simulink library "Brown_Sensors_lib"  (R2025b)
settings: Solver=VariableStepAuto  StartTime=0.0  StopTime=10.0  RelTol=1e-3
undefined symbols (not defined in the file or in its folder): default_sensor_gps_cfg, default_sensor_scalar_cfg, default_sensor_vec3_cfg, sensor_scalar_block_step, sensor_vector3_block_step
settings Model: Creator=zbrown  LastModifiedBy=zbrown

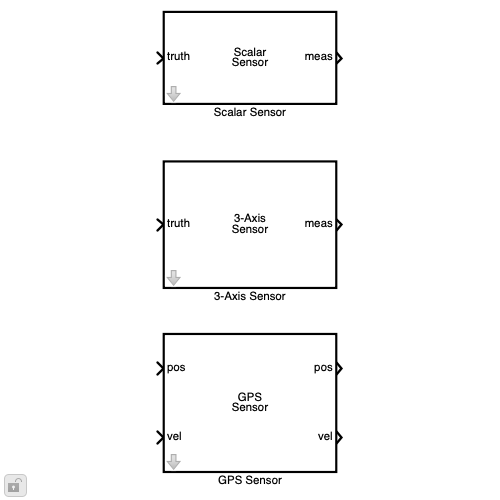
[thumbnail: Simulink's stored preview of the top-level diagram]
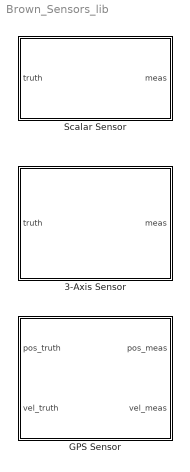
== system Brown_Sensors_lib ==
  3-Axis Sensor : Subsystem  TreatAsAtomicUnit=on  mask{cfg=default_sensor_vec3_cfg()}
      mask help: Simple reusable sensor model block.
      mask Display:
      | color('black');
      | disp('3-Axis\nSensor');
      | port_label('input',1,'truth');
      | port_label('output',1,'meas');
  GPS Sensor : Subsystem  TreatAsAtomicUnit=on  mask{cfg=default_sensor_gps_cfg()}
      mask help: Simple reusable sensor model block.
      mask Display:
      | color('black');
      | disp('GPS\nSensor');
      | port_label('input',1,'pos');
      | port_label('input',2,'vel');
      | port_label('output',1,'pos');
      | port_label('output',2,'vel');
  Scalar Sensor : Subsystem  TreatAsAtomicUnit=on  mask{cfg=default_sensor_scalar_cfg()}
      mask help: Simple reusable sensor model block.
      mask Display:
      | color('black');
      | disp('Scalar\nSensor');
      | port_label('input',1,'truth');
      | port_label('output',1,'meas');

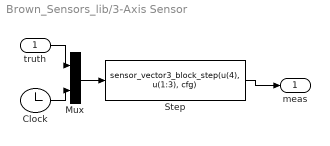
== system Brown_Sensors_lib/3-Axis Sensor ==
  truth : Inport  PortDimensions=3
  Clock : Clock
  Mux : Mux  Inputs=2
  Step : MATLABFcn  MATLABFcn=sensor_vector3_block_step(u(4), u(1:3), cfg)
  meas : Outport  PortDimensions=3
  wires:
  truth/1 -> Mux/1
  Clock/1 -> Mux/2
  Mux/1 -> Step/1
  Step/1 -> meas/1

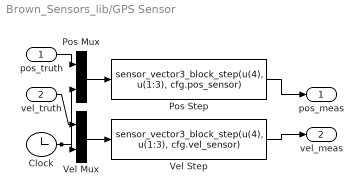
== system Brown_Sensors_lib/GPS Sensor ==
  pos_truth : Inport  PortDimensions=3
  vel_truth : Inport  Port=2  PortDimensions=3
  Clock : Clock
  Pos Mux : Mux  Inputs=2
  Pos Step : MATLABFcn  MATLABFcn=sensor_vector3_block_step(u(4), u(1:3), cfg.pos_sensor)
  Vel Mux : Mux  Inputs=2
  Vel Step : MATLABFcn  MATLABFcn=sensor_vector3_block_step(u(4), u(1:3), cfg.vel_sensor)
  pos_meas : Outport  PortDimensions=3
  vel_meas : Outport  Port=2  PortDimensions=3
  wires:
  pos_truth/1 -> Pos Mux/1
  Clock/1 -> Pos Mux/2, Vel Mux/2
  Pos Mux/1 -> Pos Step/1
  vel_truth/1 -> Vel Mux/1
  Vel Mux/1 -> Vel Step/1
  Pos Step/1 -> pos_meas/1
  Vel Step/1 -> vel_meas/1

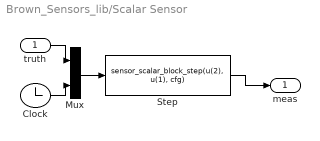
== system Brown_Sensors_lib/Scalar Sensor ==
  truth : Inport
  Clock : Clock
  Mux : Mux  Inputs=2
  Step : MATLABFcn  MATLABFcn=sensor_scalar_block_step(u(2), u(1), cfg)
  meas : Outport
  wires:
  truth/1 -> Mux/1
  Clock/1 -> Mux/2
  Mux/1 -> Step/1
  Step/1 -> meas/1
